simulink model "comparacion"  (Simulink 8.4)
settings: Solver=ode45  StartTime=0.0  StopTime=30  MaxStep=0.01  RelTol=1e-3
values from neighbouring files (symbols this model uses):
  A = XX    [codigo_Prac5.m]
  IncH2 = XX    [codigo_Prac5.m]
  IncQ = XX    [codigo_Prac5.m]
  k = As*sqrt(2*g)    [codigo_Prac5.m]
  K = XX    [codigo_Prac5.m]
  Kp_regulation = XX    [codigo_Prac5.m]
  Kp_servo = XX    [codigo_Prac5.m]
  Kp_zn = XX    [codigo_Prac5.m]
  L = XX    [codigo_Prac5.m]
  Q = 2    [codigo_Prac5.m]
  T = tau    [codigo_Prac5.m]
  Td_regulation = XX    [codigo_Prac5.m]
  Td_servo = XX    [codigo_Prac5.m]
  Td_zn = XX    [codigo_Prac5.m]
  Ti_regulation = XX    [codigo_Prac5.m]
  Ti_servo = XX    [codigo_Prac5.m]
  Ti_zn = XX    [codigo_Prac5.m]
  x0_ini = [2*XX  XX]    [codigo_Prac5.m]
settings Model: Creator=carles  LastModifiedBy=win04  CovHtmlReporting=off
settings DebuggingCC: MaxConsecutiveZCsMsg=none  FcnCallInpInsideContextMsg=EnableAllAsWarning  FrameProcessingCompatibilityMsg=error

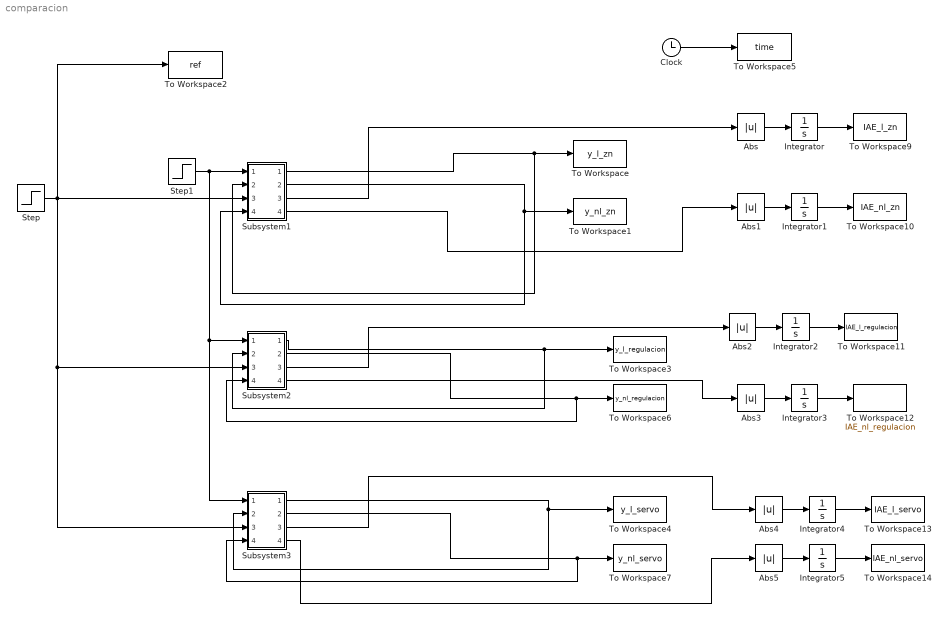
== system comparacion ==
  Abs{,1..5} (6 alike) : Abs
  Clock : Clock
  Integrator{,1..5} (6 alike) : Integrator
  Step : Step  Time=5  After=IncH2  SampleTime=0
  Step1 : Step  Time=15  After=IncQ  SampleTime=0
  Subsystem1 : Subsystem
  Subsystem2 : Subsystem
  Subsystem3 : Subsystem
  To Workspace : ToWorkspace  VariableName=y_l_zn  SampleTime=-1
  To Workspace1 : ToWorkspace  VariableName=y_nl_zn  SampleTime=-1
  To Workspace10 : ToWorkspace  VariableName=IAE_nl_zn  SampleTime=-1
  To Workspace11 : ToWorkspace  VariableName=IAE_l_regulacion  SampleTime=-1
  To Workspace12 : ToWorkspace  VariableName=IAE_nl_regulacion  SampleTime=-1
  To Workspace13 : ToWorkspace  VariableName=IAE_l_servo  SampleTime=-1
  To Workspace14 : ToWorkspace  VariableName=IAE_nl_servo  SampleTime=-1
  To Workspace2 : ToWorkspace  VariableName=ref  SampleTime=-1
  To Workspace3 : ToWorkspace  VariableName=y_l_regulacion  SampleTime=-1
  To Workspace4 : ToWorkspace  VariableName=y_l_servo  SampleTime=-1
  To Workspace5 : ToWorkspace  VariableName=time  SampleTime=-1
  To Workspace6 : ToWorkspace  VariableName=y_nl_regulacion  SampleTime=-1
  To Workspace7 : ToWorkspace  VariableName=y_nl_servo  SampleTime=-1
  To Workspace9 : ToWorkspace  VariableName=IAE_l_zn  SampleTime=-1
  wires:
  Step/1 -> Subsystem2/3(In3), Subsystem3/3(In3), Subsystem1/3(In3), To Workspace2/1
  Subsystem1/1(Out1) -> Subsystem1/2(In2), To Workspace/1
  Subsystem1/2(Out2) -> Subsystem1/4(In4), To Workspace1/1
  Step1/1 -> Subsystem1/1(In1), Subsystem3/1(In1), Subsystem2/1(In1)
  Subsystem2/1(Out1) -> Subsystem2/2(In2), To Workspace3/1
  Subsystem2/2(Out2) -> Subsystem2/4(In4), To Workspace6/1
  Abs/1 -> Integrator/1
  Integrator/1 -> To Workspace9/1
  Abs1/1 -> Integrator1/1
  Integrator1/1 -> To Workspace10/1
  Abs2/1 -> Integrator2/1
  Integrator2/1 -> To Workspace11/1
  Abs3/1 -> Integrator3/1
  Integrator3/1 -> To Workspace12/1
  Subsystem3/1(Out1) -> Subsystem3/2(In2), To Workspace4/1
  Subsystem3/2(Out2) -> Subsystem3/4(In4), To Workspace7/1
  Abs4/1 -> Integrator4/1
  Integrator4/1 -> To Workspace13/1
  Abs5/1 -> Integrator5/1
  Integrator5/1 -> To Workspace14/1
  Subsystem1/3(Out3) -> Abs/1
  Subsystem1/4(Out4) -> Abs1/1
  Subsystem2/3(Out3) -> Abs2/1
  Subsystem2/4(Out4) -> Abs3/1
  Subsystem3/3(Out3) -> Abs4/1
  Subsystem3/4(Out4) -> Abs5/1
  Clock/1 -> To Workspace5/1

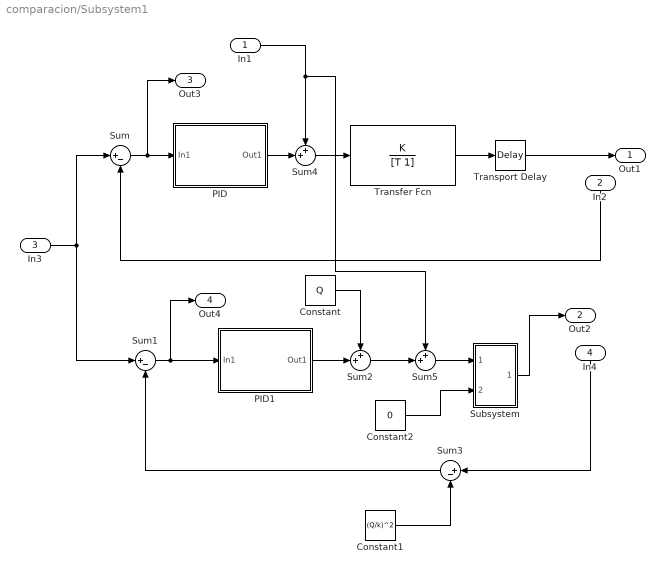
== system comparacion/Subsystem1 ==
  In1 : Inport
  In2 : Inport  Port=2
  In3 : Inport  Port=3
  In4 : Inport  Port=4
  Constant : Constant  Value=Q
  Constant1 : Constant  Value=(Q/k)^2
  Constant2 : Constant  Value=0
  PID : Subsystem
  PID1 : Subsystem
  Subsystem : Subsystem
  Sum : Sum  Inputs=|+-
  Sum1 : Sum  Inputs=|+-
  Sum2 : Sum  Inputs=++|
  Sum3 : Sum  Inputs=|+-
  Sum4 : Sum  Inputs=++|
  Sum5 : Sum  Inputs=++|
  Transfer Fcn : TransferFcn  Numerator=K  Denominator=[T 1]
  Transport Delay : TransportDelay  DelayTime=L
  Out1 : Outport
  Out2 : Outport  Port=2
  Out3 : Outport  Port=3
  Out4 : Outport  Port=4
  wires:
  In2/1 -> Sum/2
  Sum4/1 -> Transfer Fcn/1
  Subsystem/1(Out2) -> Out2/1
  PID1/1(Out1) -> Sum2/2
  In4/1 -> Sum3/1
  Constant2/1 -> Subsystem/2(In2)
  Transport Delay/1 -> Out1/1
  In1/1 -> Sum5/1, Sum4/1
  Sum2/1 -> Sum5/2
  Sum/1 -> PID/1(In1), Out3/1
  Constant/1 -> Sum2/1
  Constant1/1 -> Sum3/2
  Transfer Fcn/1 -> Transport Delay/1
  Sum3/1 -> Sum1/2
  PID/1(Out1) -> Sum4/2
  Sum5/1 -> Subsystem/1(In1)
  In3/1 -> Sum1/1, Sum/1
  Sum1/1 -> Out4/1, PID1/1(In1)

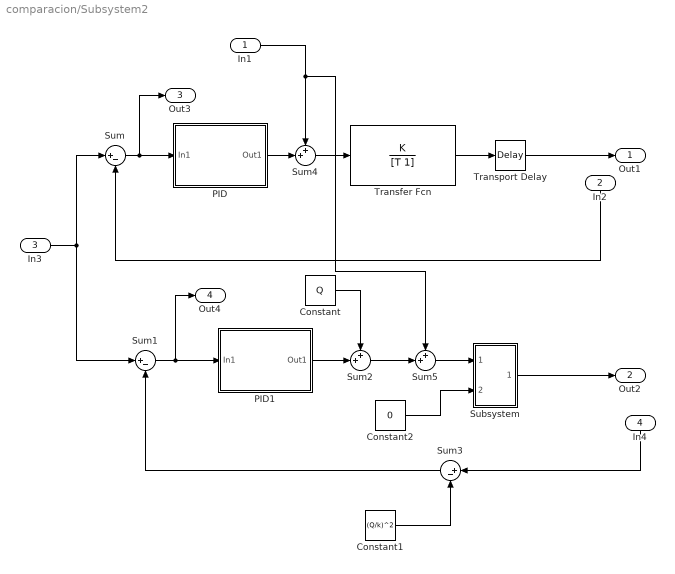
== system comparacion/Subsystem2 ==
  In1 : Inport
  In2 : Inport  Port=2
  In3 : Inport  Port=3
  In4 : Inport  Port=4
  Constant : Constant  Value=Q
  Constant1 : Constant  Value=(Q/k)^2
  Constant2 : Constant  Value=0
  PID : Subsystem
  PID1 : Subsystem
  Subsystem : Subsystem
  Sum : Sum  Inputs=|+-
  Sum1 : Sum  Inputs=|+-
  Sum2 : Sum  Inputs=++|
  Sum3 : Sum  Inputs=|+-
  Sum4 : Sum  Inputs=++|
  Sum5 : Sum  Inputs=++|
  Transfer Fcn : TransferFcn  Numerator=K  Denominator=[T 1]
  Transport Delay : TransportDelay  DelayTime=L
  Out1 : Outport
  Out2 : Outport  Port=2
  Out3 : Outport  Port=3
  Out4 : Outport  Port=4
  wires:
  In2/1 -> Sum/2
  Sum4/1 -> Transfer Fcn/1
  Subsystem/1(Out2) -> Out2/1
  PID1/1(Out1) -> Sum2/2
  In4/1 -> Sum3/1
  Constant2/1 -> Subsystem/2(In2)
  Transport Delay/1 -> Out1/1
  In1/1 -> Sum5/1, Sum4/1
  Sum2/1 -> Sum5/2
  Sum/1 -> Out3/1, PID/1(In1)
  Constant/1 -> Sum2/1
  Constant1/1 -> Sum3/2
  Transfer Fcn/1 -> Transport Delay/1
  Sum1/1 -> Out4/1, PID1/1(In1)
  Sum3/1 -> Sum1/2
  PID/1(Out1) -> Sum4/2
  Sum5/1 -> Subsystem/1(In1)
  In3/1 -> Sum1/1, Sum/1

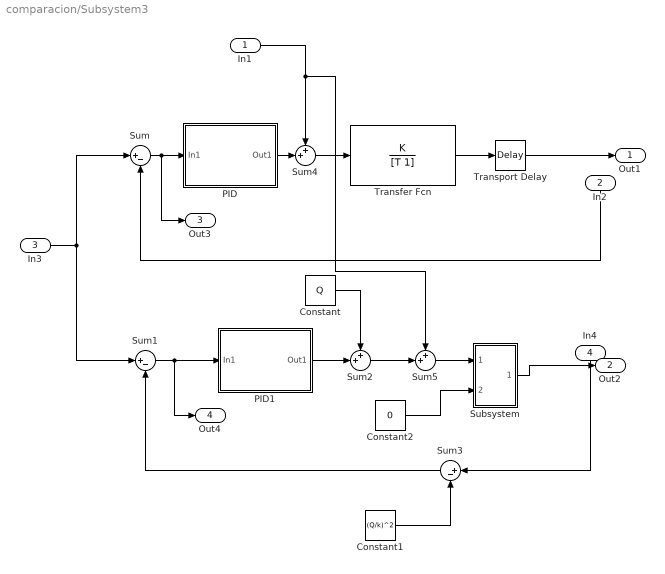
== system comparacion/Subsystem3 ==
  In1 : Inport
  In2 : Inport  Port=2
  In3 : Inport  Port=3
  In4 : Inport  Port=4
  Constant : Constant  Value=Q
  Constant1 : Constant  Value=(Q/k)^2
  Constant2 : Constant  Value=0
  PID : Subsystem
  PID1 : Subsystem
  Subsystem : Subsystem
  Sum : Sum  Inputs=|+-
  Sum1 : Sum  Inputs=|+-
  Sum2 : Sum  Inputs=++|
  Sum3 : Sum  Inputs=|+-
  Sum4 : Sum  Inputs=++|
  Sum5 : Sum  Inputs=++|
  Transfer Fcn : TransferFcn  Numerator=K  Denominator=[T 1]
  Transport Delay : TransportDelay  DelayTime=L
  Out1 : Outport
  Out2 : Outport  Port=2
  Out3 : Outport  Port=3
  Out4 : Outport  Port=4
  wires:
  In2/1 -> Sum/2
  Sum4/1 -> Transfer Fcn/1
  Subsystem/1(Out2) -> Out2/1
  PID1/1(Out1) -> Sum2/2
  In4/1 -> Sum3/1
  Constant2/1 -> Subsystem/2(In2)
  Transport Delay/1 -> Out1/1
  In1/1 -> Sum5/1, Sum4/1
  Sum2/1 -> Sum5/2
  Sum/1 -> Out3/1, PID/1(In1)
  Constant/1 -> Sum2/1
  Constant1/1 -> Sum3/2
  Transfer Fcn/1 -> Transport Delay/1
  Sum1/1 -> Out4/1, PID1/1(In1)
  Sum3/1 -> Sum1/2
  PID/1(Out1) -> Sum4/2
  Sum5/1 -> Subsystem/1(In1)
  In3/1 -> Sum1/1, Sum/1

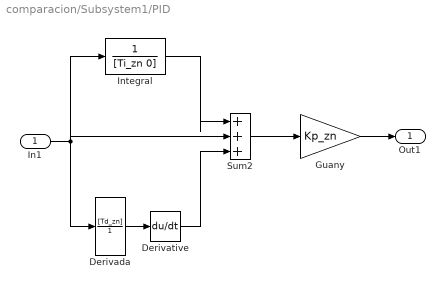
== system comparacion/Subsystem1/PID ==
  In1 : Inport
  Derivada : TransferFcn  Numerator=[Td_zn]  Denominator=[1]
  Derivative : Derivative
  Guany : Gain  Gain=Kp_zn
  Integral : TransferFcn  Denominator=[Ti_zn 0]
  Sum2 : Sum  Inputs=|+++
  Out1 : Outport
  wires:
  Guany/1 -> Out1/1
  Sum2/1 -> Guany/1
  Integral/1 -> Sum2/1
  In1/1 -> Sum2/2, Derivada/1, Integral/1
  Derivada/1 -> Derivative/1
  Derivative/1 -> Sum2/3

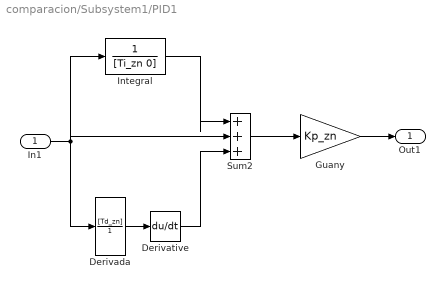
== system comparacion/Subsystem1/PID1 ==
  In1 : Inport
  Derivada : TransferFcn  Numerator=[Td_zn]  Denominator=[1]
  Derivative : Derivative
  Guany : Gain  Gain=Kp_zn
  Integral : TransferFcn  Denominator=[Ti_zn 0]
  Sum2 : Sum  Inputs=|+++
  Out1 : Outport
  wires:
  Derivative/1 -> Sum2/3
  Derivada/1 -> Derivative/1
  In1/1 -> Integral/1, Derivada/1, Sum2/2
  Integral/1 -> Sum2/1
  Sum2/1 -> Guany/1
  Guany/1 -> Out1/1

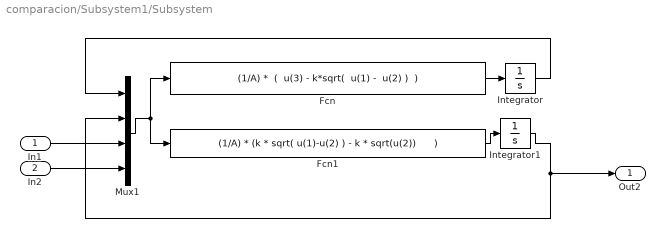
== system comparacion/Subsystem1/Subsystem ==
  In1 : Inport
  In2 : Inport  Port=2
  Fcn : Fcn  Expr="(1/A) *  (  u(3) - k*sqrt(  u(1) -  u(2) )  )"
  Fcn1 : Fcn  Expr="(1/A) * (k * sqrt( u(1)-u(2) ) - k * sqrt(u(2))      )"
  Integrator : Integrator  InitialCondition=x0_ini(1)
  Integrator1 : Integrator  InitialCondition=x0_ini(2)
  Mux1 : Mux
  Out2 : Outport
  wires:
  In1/1 -> Mux1/3
  In2/1 -> Mux1/4
  Integrator1/1 -> Out2/1, Mux1/2
  Integrator/1 -> Mux1/1
  Mux1/1 -> Fcn/1, Fcn1/1
  Fcn1/1 -> Integrator1/1
  Fcn/1 -> Integrator/1

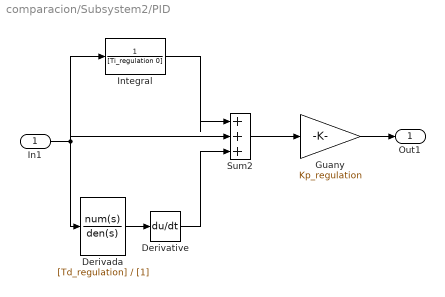
== system comparacion/Subsystem2/PID ==
  In1 : Inport
  Derivada : TransferFcn  Numerator=[Td_regulation]  Denominator=[1]
  Derivative : Derivative
  Guany : Gain  Gain=Kp_regulation
  Integral : TransferFcn  Denominator=[Ti_regulation 0]
  Sum2 : Sum  Inputs=|+++
  Out1 : Outport
  wires:
  Guany/1 -> Out1/1
  Sum2/1 -> Guany/1
  Integral/1 -> Sum2/1
  In1/1 -> Sum2/2, Derivada/1, Integral/1
  Derivada/1 -> Derivative/1
  Derivative/1 -> Sum2/3

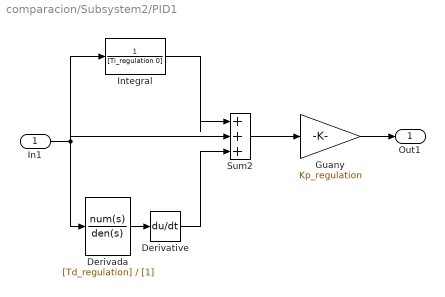
== system comparacion/Subsystem2/PID1 ==
  In1 : Inport
  Derivada : TransferFcn  Numerator=[Td_regulation]  Denominator=[1]
  Derivative : Derivative
  Guany : Gain  Gain=Kp_regulation
  Integral : TransferFcn  Denominator=[Ti_regulation 0]
  Sum2 : Sum  Inputs=|+++
  Out1 : Outport
  wires:
  Derivative/1 -> Sum2/3
  Derivada/1 -> Derivative/1
  In1/1 -> Integral/1, Derivada/1, Sum2/2
  Integral/1 -> Sum2/1
  Sum2/1 -> Guany/1
  Guany/1 -> Out1/1

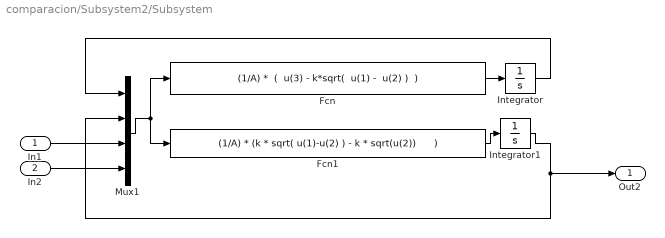
== system comparacion/Subsystem2/Subsystem ==
  In1 : Inport
  In2 : Inport  Port=2
  Fcn : Fcn  Expr="(1/A) *  (  u(3) - k*sqrt(  u(1) -  u(2) )  )"
  Fcn1 : Fcn  Expr="(1/A) * (k * sqrt( u(1)-u(2) ) - k * sqrt(u(2))      )"
  Integrator : Integrator  InitialCondition=x0_ini(1)
  Integrator1 : Integrator  InitialCondition=x0_ini(2)
  Mux1 : Mux
  Out2 : Outport
  wires:
  In1/1 -> Mux1/3
  In2/1 -> Mux1/4
  Integrator1/1 -> Out2/1, Mux1/2
  Integrator/1 -> Mux1/1
  Mux1/1 -> Fcn/1, Fcn1/1
  Fcn1/1 -> Integrator1/1
  Fcn/1 -> Integrator/1

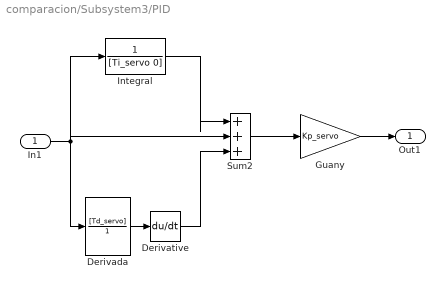
== system comparacion/Subsystem3/PID ==
  In1 : Inport
  Derivada : TransferFcn  Numerator=[Td_servo]  Denominator=[1]
  Derivative : Derivative
  Guany : Gain  Gain=Kp_servo
  Integral : TransferFcn  Denominator=[Ti_servo 0]
  Sum2 : Sum  Inputs=|+++
  Out1 : Outport
  wires:
  Guany/1 -> Out1/1
  Sum2/1 -> Guany/1
  Integral/1 -> Sum2/1
  In1/1 -> Sum2/2, Derivada/1, Integral/1
  Derivada/1 -> Derivative/1
  Derivative/1 -> Sum2/3

== system comparacion/Subsystem3/PID1 ==
  In1 : Inport
  Derivada : TransferFcn  Numerator=[Td_servo]  Denominator=[1]
  Derivative : Derivative
  Guany : Gain  Gain=Kp_servo
  Integral : TransferFcn  Denominator=[Ti_servo 0]
  Sum2 : Sum  Inputs=|+++
  Out1 : Outport
  wires:
  Derivative/1 -> Sum2/3
  Derivada/1 -> Derivative/1
  In1/1 -> Integral/1, Derivada/1, Sum2/2
  Integral/1 -> Sum2/1
  Sum2/1 -> Guany/1
  Guany/1 -> Out1/1

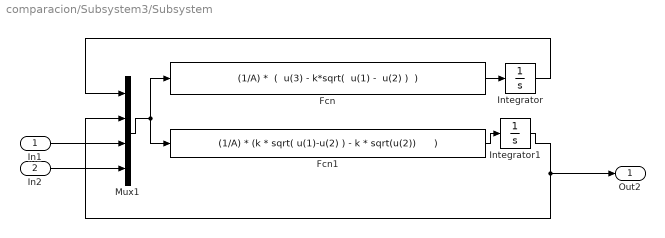
== system comparacion/Subsystem3/Subsystem ==
  In1 : Inport
  In2 : Inport  Port=2
  Fcn : Fcn  Expr="(1/A) *  (  u(3) - k*sqrt(  u(1) -  u(2) )  )"
  Fcn1 : Fcn  Expr="(1/A) * (k * sqrt( u(1)-u(2) ) - k * sqrt(u(2))      )"
  Integrator : Integrator  InitialCondition=x0_ini(1)
  Integrator1 : Integrator  InitialCondition=x0_ini(2)
  Mux1 : Mux
  Out2 : Outport
  wires:
  In1/1 -> Mux1/3
  In2/1 -> Mux1/4
  Integrator1/1 -> Out2/1, Mux1/2
  Integrator/1 -> Mux1/1
  Mux1/1 -> Fcn/1, Fcn1/1
  Fcn1/1 -> Integrator1/1
  Fcn/1 -> Integrator/1
